simulink model "LQR_CONTROL2"  (R2015a)
settings: Solver=ode45  StartTime=0.0  StopTime=10.0  RelTol=1e-3
undefined symbols (not defined in the file): A_m, B_m, C_m, D_m, K_1, K_2, K_3
settings Model: Creator=vinay  LastModifiedBy=vinay

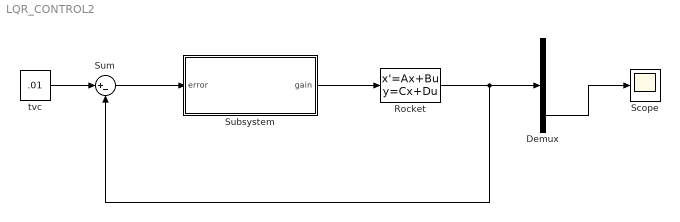
== system LQR_CONTROL2 ==
  Demux : Demux  Outputs=3
  Rocket : StateSpace  A=A_m  B=B_m  C=C_m  D=D_m  X0=[0.2;0;0]
  Scope : Scope
  Subsystem : Subsystem
  Sum : Sum  Inputs=|+-
  tvc : Constant  Value=.01
  wires:
  tvc/1 -> Sum/1
  Rocket/1 -> Demux/1, Sum/2
  Sum/1 -> Subsystem/1(error)
  Subsystem/1(gain) -> Rocket/1
  Demux/3 -> Scope/1

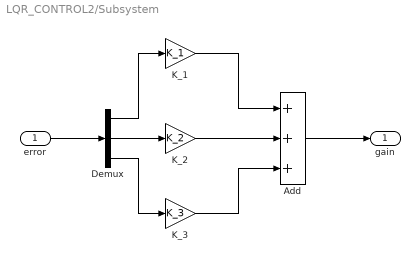
== system LQR_CONTROL2/Subsystem ==
  error : Inport
  Add : Sum  Inputs=+++
  Demux : Demux  Outputs=3
  K_1 : Gain  Gain=K_1
  K_2 : Gain  Gain=K_2
  K_3 : Gain  Gain=K_3
  gain : Outport
  wires:
  Add/1 -> gain/1
  Demux/1 -> K_1/1
  K_1/1 -> Add/1
  K_2/1 -> Add/2
  K_3/1 -> Add/3
  error/1 -> Demux/1
  Demux/3 -> K_3/1
  Demux/2 -> K_2/1
